simulink model "OLD_Master"  (R2023b)
settings: Solver=VariableStepAuto  StartTime=0.0  StopTime=inf  RelTol=1e-3
values from neighbouring files (symbols this model uses):
  Analog_Left_X = Simulink.BusElement    [globalStruct.m]
  Analog_Left_Y = Simulink.BusElement    [globalStruct.m]
  Battery_Level = Simulink.BusElement    [globalStruct.m]
  Communication = Simulink.BusElement    [globalStruct.m]
  Cross = Simulink.BusElement    [globalStruct.m]
  Square = Simulink.BusElement    [globalStruct.m]
undefined symbols (not defined in the file or in its folder): Distance_Left, Distance_Middle, Distance_Right, Dpad_Left, Dpad_Right, Encoder
settings Model: Creator=sabat  LastModifiedBy=sabat
settings OptimizationCC: DefaultParameterBehavior=Inlined  EnhancedBackFolding=on  PassReuseOutputArgsAs=Individual arguments  ZeroExternalMemoryAtStartup=off  ZeroInternalMemoryAtStartup=off  OptimizeBlockOrder=speed  DifferentSizesBufferReuse=on  OptimizationCustomize=off  EfficientTunableParamExpr=on
settings DebuggingCC: ParameterTunabilityLossMsg=error
settings SFSimCC: MATLABDynamicMemAlloc=off
settings RTWCC: Description=Embedded Coder  SystemTargetFile=ert.tlc  TemplateMakefile=ert_default_tmf
settings CodeAppCC: ForceParamTrailComments=on  IgnoreCustomStorageClasses=off  OperatorAnnotations=on  SimulinkDataObjDesc=on  SFDataObjDesc=on  InsertBlockDesc=on
settings ERTTargetCC: TargetLangStandard=C99 (ISO)  GenerateSampleERTMain=on  InlinedParameterPlacement=NonHierarchical  ERTCustomFileTemplate=example_file_process.tlc

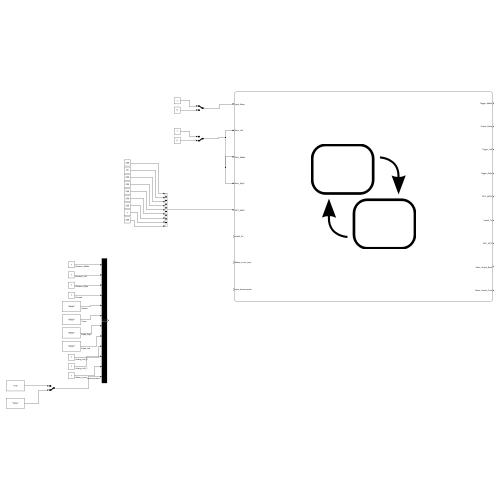
[thumbnail: Simulink's stored preview of the top-level diagram]
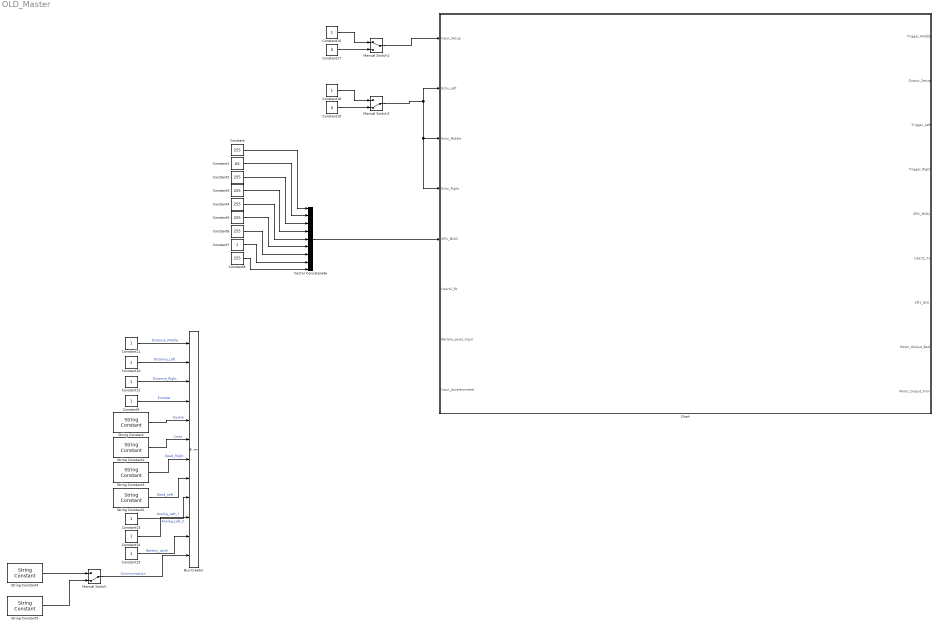
== system OLD_Master ==
  Bus Creator : BusCreator  Inputs=Distance_Middle,Distance_Left,Distance_Right,Encoder,Square,Cross,Dpad_Right,Dpad_Left,Analog_Left_X,Analog_Left_Y,Battery_Level,Communication  OutDataTypeStr=Bus: global_var
  Chart : Stateflow chart  TreatAsAtomicUnit=on
  Constant{,2..6,8} (7 alike) : Constant  Value=255
  Constant1 : Constant  Value=65
  Constant{7,9..16,18} (10 alike) : Constant
  Constant17 : Constant  Value=0
  Constant19 : Constant  Value=0
  Manual Switch : ManualSwitch  CurrentSetting=0
  Manual Switch1 : ManualSwitch
  Manual Switch2 : ManualSwitch  CurrentSetting=0
  String Constant{,1..3} (4 alike) : StringConstant
  String Constant4 : StringConstant  String="\"1/2\""
  String Constant5 : StringConstant  String="\"Alive\""
  Vector Concatenate : Concatenate  NumInputs=9
  wires:
  Constant/1 -> Vector Concatenate/1
  Constant1/1 -> Vector Concatenate/2
  Constant2/1 -> Vector Concatenate/3
  Constant3/1 -> Vector Concatenate/4
  Constant4/1 -> Vector Concatenate/5
  Constant5/1 -> Vector Concatenate/6
  Constant6/1 -> Vector Concatenate/7
  Constant7/1 -> Vector Concatenate/8
  Constant8/1 -> Vector Concatenate/9
  Vector Concatenate/1 -> Chart/5(SPI1_MISO)
  Constant11/1 -> Bus Creator/1  "Distance_Middle"
  Constant10/1 -> Bus Creator/2  "Distance_Left"
  Constant12/1 -> Bus Creator/3  "Distance_Right"
  Constant9/1 -> Bus Creator/4  "Encoder"
  String Constant/1 -> Bus Creator/5  "Square"
  String Constant1/1 -> Bus Creator/6  "Cross"
  String Constant3/1 -> Bus Creator/7  "Dpad_Right"
  String Constant2/1 -> Bus Creator/8  "Dpad_Left"
  Constant13/1 -> Bus Creator/9  "Analog_Left_X"
  Constant14/1 -> Bus Creator/10  "Analog_Left_Y"
  Constant15/1 -> Bus Creator/11  "Battery_Level"
  Manual Switch/1 -> Bus Creator/12  "Communication"
  String Constant5/1 -> Manual Switch/2
  Manual Switch1/1 -> Chart/1(Input_Setup)
  Constant16/1 -> Manual Switch1/1
  Constant17/1 -> Manual Switch1/2
  Constant18/1 -> Manual Switch2/1
  Constant19/1 -> Manual Switch2/2
  Manual Switch2/1 -> Chart/4(Echo_Right), Chart/3(Echo_Middle), Chart/2(Echo_Left)
  String Constant4/1 -> Manual Switch/1

== stateflow chart OLD_Master/Chart ==
  state Setup_State
    state Send_My_Part_Setup
      Usart2_Tx.Communication="Alive";
    state Off
      Output_Setup=1;
      Usart2_Tx.Communication="0";
    state On
      en: send(Read_Ultrasounds,Setup_State);
    (default) -> Send_My_Part_Setup
    Send_My_Part_Setup -> Off : [Usart2_Rx.Communication == "Alive"]
    Off -> On : [Input_Setup == 1]
  state Read_Ultrasounds_State
    state Logic [parallel]
      settings: executionOrder=1
      state Sensor_Not_Read
      state Sensor_Read
      (default) -> Read_Ultrasounds_State.Logic.Sensor_Not_Read
      Read_Ultrasounds_State.Logic.Sensor_Not_Read -> Read_Ultrasounds_State.Logic.Sensor_Read : [after(1,Ultrasound_Read_Middle) && after(1,Ultrasound_Read_Left) && after(1,Ultrasound_Read_Right) && after(1,Controller_Read) && after(Ultrasounds_Deadline, msec)]{send(Check_Danger, Read_Ultrasounds_State)}
    state Ultrasound_Middle [parallel]
      settings: executionOrder=2
      state Trigger_on
        Trigger_Middle=1;
      state Wait
        Trigger_Middle=0;
      state End
      state Counting
        en,du: y_Middle =temporalCount(usec);
      (default) -> Read_Ultrasounds_State.Ultrasound_Middle.Trigger_on
      Read_Ultrasounds_State.Ultrasound_Middle.Trigger_on -> Read_Ultrasounds_State.Ultrasound_Middle.Wait : [after(10, usec)]
      Read_Ultrasounds_State.Ultrasound_Middle.Wait -> Read_Ultrasounds_State.Ultrasound_Middle.Counting : [after(60,msec) && Echo_Middle == 1]
      Read_Ultrasounds_State.Ultrasound_Middle.Counting -> Read_Ultrasounds_State.Ultrasound_Middle.End : [Echo_Left == 0]{Global_Struct.Distance_Middle= y_Middle*0.017;send(Ultrasound_Read_Middle,Read_Ultrasounds_State.Logic);}
    state Ultrasound_Left [parallel]
      settings: executionOrder=3
      state Trigger_on
        Trigger_Left=1;
      state Wait
        Trigger_Left=0;
      state Counting
        en,du: y_Left =temporalCount(usec);
      state End
      (default) -> Read_Ultrasounds_State.Ultrasound_Left.Trigger_on
      Read_Ultrasounds_State.Ultrasound_Left.Trigger_on -> Read_Ultrasounds_State.Ultrasound_Left.Wait : [after(10, usec)]
      Read_Ultrasounds_State.Ultrasound_Left.Wait -> Read_Ultrasounds_State.Ultrasound_Left.Counting : [after(60,msec) && Echo_Left == 1]
      Read_Ultrasounds_State.Ultrasound_Left.Counting -> Read_Ultrasounds_State.Ultrasound_Left.End : [Echo_Left == 0]{Global_Struct.Distance_Left= y_Left*0.017;send(Ultrasound_Read_Left,Read_Ultrasounds_State.Logic);}
    state Ultrasound_Right [parallel]
      settings: executionOrder=4
      state Trigger_on
        Trigger_Right=1;
      state Wait
        Trigger_Right=0;
      state Counting
        en,du: y_Right =temporalCount(usec);
      state End
      (default) -> Read_Ultrasounds_State.Ultrasound_Right.Trigger_on
      Read_Ultrasounds_State.Ultrasound_Right.Trigger_on -> Read_Ultrasounds_State.Ultrasound_Right.Wait : [after(10, usec)]
      Read_Ultrasounds_State.Ultrasound_Right.Wait -> Read_Ultrasounds_State.Ultrasound_Right.Counting : [after(60,msec) && Echo_Right == 1]
      Read_Ultrasounds_State.Ultrasound_Right.Counting -> Read_Ultrasounds_State.Ultrasound_Right.End : [Echo_Right == 0]{Global_Struct.Distance_Right= y_Right*0.017;send(Ultrasound_Read_Right,Read_Ultrasounds_State.Logic);}
  state Check_Danger_State
    state Check
      Distance_Middle_Err=0;
      Distance_Left_Err = 0;
      Distance_Right_Err = 0;
      if Global_Struct.Distance_Middle <=0.7
      %fermati pesante
      Distance_Middle_Err=1;
      elseif  Global_Struct.Distance_Middle  >0.7 && Global_Struct.Distance_Middle  <3
      %fermati lieve e
      %potenzialemte parti dopo
      Distance_Middle_Err=2;
      end
      if Global_Struct.Distance_Left <=0.7
      %fermati pesante
      Distance_Left_Err=1;
      elseif (Global_Struct.Distance_Left  >0.7 && Global_Struct.Distance_Left  <3)
      %fermati lieve e
      %potenzialemte parti dopo
      Distance_Left_Err=2;
      end
      if Global_Struct.Distance_Right <=0.7
      %fermati pesante
      Distance_Right_Err=1;
      elseif Global_Struct.Distance_Right  >0.7 && Global_Struct.Distance_Right  <3
      %fermati lieve e
      %potenzialemte parti dopo
      Distance_Right_Err=2;
      end
    state Check_End
    (default) -> Check
    Check -> Check_End [order 1] : [Distance_Middle_Err ~= 0 || Distance_Left_Err ~= 0 || DIstance_Right_Err ~= 0]{send(Outputs, Check_Danger_State)}
    Check -> Check_End [order 2] : [Distance_Middle_Err == 0 && Distance_Left_Err == 0 && Distance_Right_Err && 0]{ send(Read_Other_Inputs, Check_Danger_State)}
  state Read_Other_Inputs_State
    state Logic [parallel]
      settings: executionOrder=1
      state Sensor_Not_Read
      state Sensor_Read
      (default) -> Read_Other_Inputs_State.Logic.Sensor_Not_Read
      Read_Other_Inputs_State.Logic.Sensor_Not_Read -> Read_Other_Inputs_State.Logic.Sensor_Read : [ after(1,Controller_Read) && after(Inputs_Deadline, msec)]{send(Processing, Read_Other_Inputs_State)}
    state Accelerometer [parallel]
      Global_Struct = Input_Accelerometer;
      settings: executionOrder=3
    state Controller [parallel]
      settings: executionOrder=2
      state Controller_Read
        SPI1_NCC=0;
        SPI1_MOSI= [1 66];
        Read=SPI1_MISO;
        SPI1_NCC=1;
        done=0;
        if Read(1) == 255 && Read(2) == 255 && Read(3) == 255 && Read(4) == 255 && Read(5) == 255 && Read(6) == 255 && Read(7) == 255 && Read(8) == 255 && Read(9) == 255
        Controller_Ok = 0;
        else
        Controller_Ok=1;
        end
      state Digital
        Global_Struct.Square = "1";
        Global_Struct.Cross = "1";
        Global_Struct.Dpad_Right = "1";
        Global_Struct.Dpad_Left = "1";
        done=1;
      state Analog
        %Da verificare i byte se sono corretti
        Global_Struct.Analog_Left_X = Read(6);
        Global_Struct.Analog_Left_Y = Read(7);
        done=1;
      state End
      (default) -> Controller_Read
      Controller_Read -> Digital [order 1] : [Read(2) == 65]
      Controller_Read -> Analog [order 2] : [Read(2) == 115]
      Digital -> Read_Other_Inputs_State.Controller.End : [done == 1]{send(Controller_Read,Read_Inputs_State.Logic);}
      Analog -> Read_Other_Inputs_State.Controller.End : [done==1]{send(Controller_Read,Read_Inputs_State.Logic);}
  state Processing_State
    state Send_My_Part
      en: Global_Struct.Communication="1/2";
      en: Usart2_Tx=Global_Struct;
      en: Slave_Communication=0;
    state Receive_Slave_Part
      en:Usart2_Tx.Communication="0";
      %Faccio calcoli e se non mi trovo
      %devo richiedere reinvio il mex
    state Go_Other_State
    state Send_Yes
      Usart2_Tx.Communication="Yes";
    state Timer
    Send_My_Part -> Send_My_Part [order 2] : [after(TIMEOUT,msec)]
    (default) -> Send_My_Part [order 1]
    Send_My_Part -> Receive_Slave_Part [order 1] : [Usart2_Rx.Communication == "1/2"]
    Receive_Slave_Part -> Send_My_Part [order 1] : [Usart2_Rx.Communication ~= "1/2" ]
    Receive_Slave_Part -> Send_Yes [order 2] : [Usart2_Rx.Communication == "1/2"]
    Send_Yes -> Send_Yes [order 2] : [after(timeout,msec)]
    Send_Yes -> Go_Other_State [order 1] : [Usart2_Rx.Communication == "ACK"]{Slave_Communication=1;
        | Usart2_Tx.Communication="0";}
    Timer -> Timer : [after(Processing_Deadline, msec)]{send(Outputs,Processing_State)}
    (default) -> Timer [order 2]
  state Outputs_State
    state Check_input
      state Check_Motor_Response
        %devo verificare che i motori
        %rispondano leggere da encoder
        %Idea: vedere ultimo comando
        %inviato = direzione letta
        ALL_OK= 0
      state Start
        ALL_OK = 0;
        if Distance_Middle_Err ~= 0 || Distance_Left_Err ~= 0 || Distance_Right_Err ~= 0
        ALL_OK = 2;
        else
        ALL_OK = 0;
        end
      state Check_PSX_Alive
        if Controller_Ok == 0
        ALL_OK=2;
        else
        ALL_OK=0;
        end
      state Check_Board
        if Slave_Communication ==1
        Check_OK=0;
        else
        ALL_OK=1;
        end
      state Check_Battery
        %devo verificare la batteria
        if Global_Struct.Battery_Levele < 23
        ALL_OK=2
        else
        ALL_OK=0
        end
      state Check_Temperature
        %devo verificare la temperatura
        if Global_Struct.Battery_Temperature > 50
        ALL_OK=2;
        else
        ALL_OK=0;
        end
      Check_PSX_Alive -> Check_input [order 2] : [ALL_OK == 2]
      Check_Motor_Response -> Check_input [order 2] : [ALL_OK == 2]
      (default) -> Start
      Check_PSX_Alive -> Check_Motor_Response [order 1] : [ALL_OK == 0]
      Check_Motor_Response -> Check_Temperature [order 1] : [ALL_OK == 2]
      Start -> Check_PSX_Alive [order 2] : [ALL_OK == 0]
      Start -> Check_input [order 1] : [ALL_OK == 2]
      Check_Board -> Check_input
      Check_Battery -> Check_Board [order 2] : [ALL_OK == 0]
      Check_Temperature -> Check_Battery [order 2] : [ALL_OK ==0]
      Check_Temperature -> Check_input [order 1] : [ALL_OK==2]
      Check_Battery -> Check_input [order 1] : [ALL_OK == 2]
    state Emergency_Stop
      %%Non mettere 0 ma puoi anche andare in senso opposto al movimento per fermarti prima
      Motor_Output_Front= 0;
      Motor_Output_Back= 0;
    state Drive
      %In partiolare il valore da impartire ai motori differisce nei due driver perchè abbiamo che quando giriamo il verso e
      % intensità sono discordi, QUINDI VALORI SEGUENTI NON VERITIERI
      Motor_Output_Front= Global_Struct.Analog_Left_X;
      Motor_Output_Back= Global_Struct.Analog_Left_X;
    state Degradated_Drive
      Disable_Slave = 1;
      Motor_Output_Front= Global_Struct.Analog_Left_X%120;
      Motor_Output_Back= Global_Struct.Analog_Left_X%120;
    Check_input -> Emergency_Stop [order 3] : [ALL_OK == 2]
    (default) -> Check_input
    Check_input -> Drive [order 2] : [ALL_OK== 0]
    Check_input -> Degradated_Drive [order 1] : [ALL_OK == 1]
  Outputs_State -> Read_Ultrasounds_State : [Read_Ultrasounds]
  Check_Danger_State -> Outputs_State [order 1] : Outputs
  (default) -> Setup_State
  Check_Danger_State -> Read_Other_Inputs_State [order 2] : [Read_Other_Inputs]
  Read_Other_Inputs_State -> Processing_State : [Processing]
  Processing_State -> Outputs_State : [Outputs]
  Setup_State -> Read_Ultrasounds_State : [Read_Ultrasounds]
  Read_Ultrasounds_State -> Check_Danger_State : [Check_Danger]
  data: y_Middle local double size=1; Trigger_Middle output double size=1; Input_Setup input double size=1; Output_Setup output double size=1; Trigger_Left output double size=1; Echo_Left input double size=1; y_Left local double size=1; Echo_Middle input double size=1; Echo_Right input double size=1; SPI1_MISO input double size=9; Trigger_Right output double size=1; y_Right local double size=1; TIMEOUT local double size=1 =15; timeout local double size=1 =15; Deadline_Processing local double size=1; Counting_Deadline local double size=1; SPI1_MOSI output double size=[1 2]; Usart2_Tx output Bus: global_var size=1; Usart2_Rx input Bus: global_var size=1; App_Usart2_Tx local string; Battery_Level_Input input double size=1; SPI1_NCC output size=1; Read local double size=9; Global_Struct local Bus: global_var size=1; done local; ALL_OK local; Inputs_Deadline local; Input_Accelerometer input; DIstance_Right_Err local; Processing_Deadline local; Disable_Slave local; Motor_Output_Back output; Motor_Output_Front output; Slave_Communication local; Distance_Right_Err local; Distance_Middle_Err local; Distance_Left_Err local; Controller_Ok local; Ultrasounds_Deadline local
  events: Processing local FUNCTION_CALL_EVENT; Read_Inputs local FUNCTION_CALL_EVENT; Ultrasound_Read_Middle local FUNCTION_CALL_EVENT; Outputs local FUNCTION_CALL_EVENT; Ultrasound_Read_Left local FUNCTION_CALL_EVENT; Ultrasound_Read_Right local FUNCTION_CALL_EVENT; Controller_Read local FUNCTION_CALL_EVENT; Check_Danger local FUNCTION_CALL_EVENT; Read_Other_Inputs local FUNCTION_CALL_EVENT; Read_Ultrasounds local FUNCTION_CALL_EVENT
